simulink subsystem "Actionneur_lineaire"  (R2019b)
settings: Solver=VariableStepAuto  StartTime=0.0  StopTime=10.0  RelTol=1e-3
values from neighbouring files (symbols this model uses):
  B_bobine = 0.1128    [default_design_data.mat]    (also in dict.sldd)
  K_e = 0.9495    [default_design_data.mat]    (also in dict.sldd)
  L_bobine = 212    [default_design_data.mat]    (also in dict.sldd = 212.0)
  N_bobine = 66    [default_design_data.mat]    (also in dict.sldd = 1000.0)
  R_bobine = 1.424    [default_design_data.mat]    (also in dict.sldd)
  r_bobine = 0.0203    [default_design_data.mat]    (also in dict.sldd)
  R_eq = 1.1    [default_design_data.mat]    (also in dict.sldd)
settings Model: Creator=frfoc1  LastModifiedBy=freud

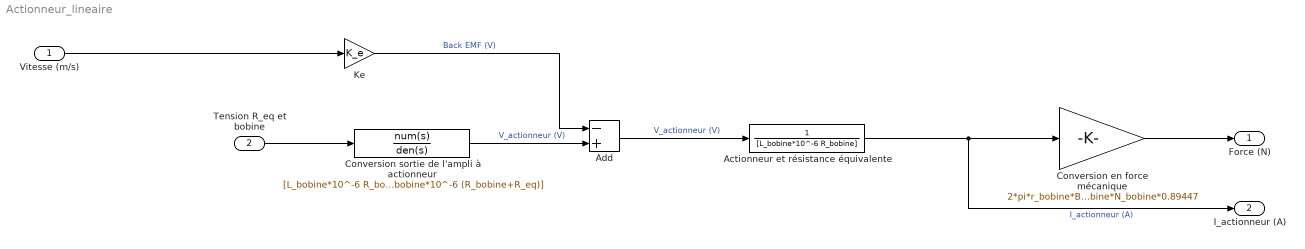
== system Actionneur_lineaire ==
  Vitesse (m/s) : Inport
  Tension R_eq et bobine : Inport  Port=2
  Actionneur et résistance équivalente : TransferFcn  Denominator=[L_bobine*10^-6 R_bobine]
  Add : Sum  Inputs=-+
  Conversion en force mécanique : Gain  Gain=2*pi*r_bobine*B_bobine*N_bobine*0.89447
  Conversion sortie de l'ampli à actionneur : TransferFcn  Numerator=[L_bobine*10^-6 R_bobine]  Denominator=[L_bobine*10^-6 (R_bobine+R_eq)]
  Ke : Gain  Gain=K_e
  Force (N) : Outport
  I_actionneur (A) : Outport  Port=2
  wires:
  Add/1 -> Actionneur et résistance équivalente/1  "V_actionneur (V)"
  Conversion sortie de l'ampli à actionneur/1 -> Add/2  "V_actionneur (V)"
  Conversion en force mécanique/1 -> Force (N)/1
  Actionneur et résistance équivalente/1 -> Conversion en force mécanique/1, I_actionneur (A)/1  "I_actionneur (A)"
  Ke/1 -> Add/1  "Back EMF (V)"
  Vitesse (m/s)/1 -> Ke/1
  Tension R_eq et bobine/1 -> Conversion sortie de l'ampli à actionneur/1
